simulink model "gm_stream_adaptation_model_fil"  (R2020b)
settings: Solver=FixedStepDiscrete  StartTime=0.0  StopTime=2  RelTol=1e-3
values from neighbouring files (symbols this model uses):
  frame = [frame zeros(num_of_pad_bits, 1)]    [pad_and_scramble.m]    (also in pad_and_scramble_test.m = randi([0 1], Kbch, 1); scrambler.m = in_frame)
libraries: simulink x3, hdlsllib x2, whdlio x1, fillib x1
settings Model: Creator=wardo  LastModifiedBy=EFlores
settings DataIOCC: LimitDataPoints=on  SaveOutput=off  SaveTime=off
settings OptimizationCC: BlockReduction=off  ConditionallyExecuteInputs=off  DefaultParameterBehavior=Inlined  LifeSpan=inf
settings DebuggingCC: AlgebraicLoopMsg=error  InheritedTsInSrcMsg=none  SingleTaskRateTransMsg=error  AllowSymbolicDim=off  StrictBusMsg=ErrorOnBusTreatedAsVector  SFUnexpectedBacktrackingDiag=warning  SFNoUnconditionalDefaultTransitionDiag=warning  SFExecutionAtInitializationDiag=none  ArithmeticOperatorsInVariantConditions=warning
settings HardwareCC: ProdBitPerPointer=32  ProdBitPerSizeT=32  ProdBitPerPtrDiffT=32  ProdLargestAtomicFloat=None  ProdIntDivRoundTo=Undefined  ProdEndianess=Unspecified  ProdWordSize=32  ProdHWDeviceType=ASIC/FPGA->ASIC/FPGA  ProdEqTarget=off
settings SFSimCC: SimUseLocalCustomCode=off  CustomCodeUndefinedFunction=UseInterfaceOnly
settings RTWCC: RTWUseLocalCustomCode=off
settings CodeAppCC: StateflowObjectComments=on
settings GRTTargetCC: TargetLangStandard=C89/C90 (ANSI)
settings ConfigComp: CovScope=ReferencedModels  CovMetricSettings=dw  CovSaveCumulativeToWorkspaceVar=on  CovSaveSingleToWorkspaceVar=on  CovExternalEMLEnable=off  CovSFcnEnable=off

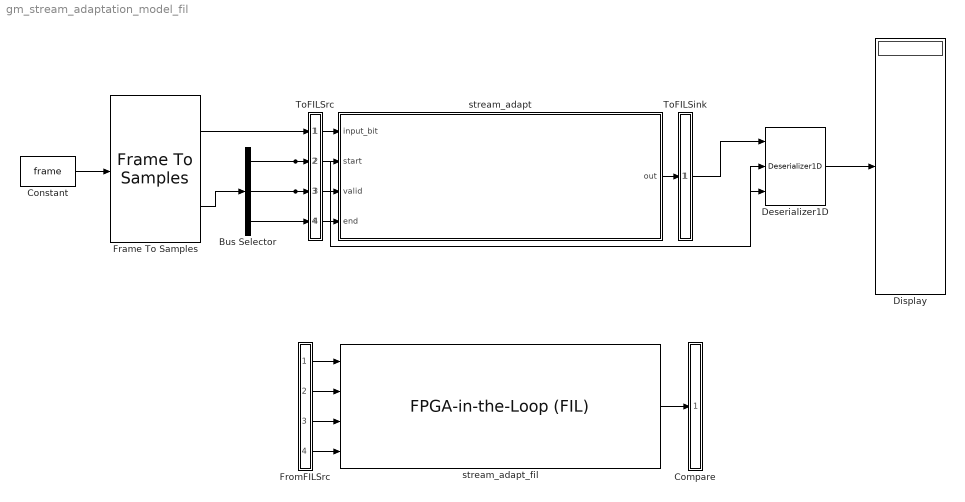
== system gm_stream_adaptation_model_fil ==
  Bus Selector : BusSelector  OutputSignals=start,valid,end
  Compare : Subsystem
      mask Display: disp('')
  Constant : Constant  Value=frame  OutDataTypeStr=fixdt(1,16)  SampleTime=1
  Deserializer1D : hdlsllib/HDL Operations/Deserializer1D  Ratio=48408  IdleCycles=0  InitialCondition=0  startIn=on  validIn=on  validOut=off  inputDataDimensions=-1  inputSampleTime=-1  inputSignalType=auto
      settings: SourceProductBaseCode=SL
  Display : Display
  Frame To Samples : whdlio/Frame To Samples  InterSampleIdleCycles=0  InterFrameIdleCycles=0  OutputSize=1  InterleaveSamples=off
      settings: SourceProductBaseCode=LH
  FromFILSrc : Subsystem
      mask Display: disp('')
  ToFILSink : Subsystem
      mask Display: disp('')
  ToFILSrc : Subsystem
      mask Display: disp('')
  stream_adapt : Subsystem
  stream_adapt_fil : fillib/FPGA-in-the-Loop (FIL)  ForceInterfaceUpdate=0.85357
      settings: SourceProductBaseCode=ES,HD
  wires:
  Constant/1 -> Frame To Samples/1
  Frame To Samples/2 -> Bus Selector/1
  Bus Selector/1 -> Deserializer1D/2, ToFILSrc/2(in2)
  Bus Selector/2 -> Deserializer1D/3, ToFILSrc/3(in3)
  Deserializer1D/1 -> Display/1
  ToFILSrc/1(out1) -> stream_adapt/1(input_bit)
  ToFILSrc/2(out2) -> stream_adapt/2(start)
  ToFILSrc/3(out3) -> stream_adapt/3(valid)
  ToFILSrc/4(out4) -> stream_adapt/4(end)
  stream_adapt/1(out) -> ToFILSink/1(in1)
  Frame To Samples/1 -> ToFILSrc/1(in1)
  Bus Selector/3 -> ToFILSrc/4(in4)
  ToFILSink/1(out1) -> Deserializer1D/1
  FromFILSrc/1(out1) -> stream_adapt_fil/1
  FromFILSrc/2(out2) -> stream_adapt_fil/2
  FromFILSrc/3(out3) -> stream_adapt_fil/3
  FromFILSrc/4(out4) -> stream_adapt_fil/4
  stream_adapt_fil/1 -> Compare/1(in1)

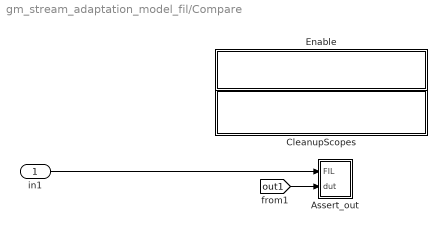
== system gm_stream_adaptation_model_fil/Compare ==
  in1 : Inport
  Assert_out : Subsystem
  CleanupScopes : Subsystem
      settings: OpenFcn=|
      | blkName = gcb; %self block
      | idx = regexp(blkName, '/CleanupScopes$', 'once');
      | blkParent = blkName(1:idx-1);
      | blks=find_system(blkParent, 'LookUnderMasks', 'all','blocktype', 'Scope');
      | for itr = 1:length(blks)
      | 	 hScopeCfg = get_param(blks{itr},'ScopeConfiguration');
      | 	 hScopeCfg.Visible = ~ hScopeCfg.Visible;
      | end
      | drawnow;
      mask Display: fprintf(message('hdlcoder:cosim:vnl_dblclick').getString());
  Enable : Subsystem
      settings: OpenFcn=|
      | blkName = gcb;
      | idx = regexp(blkName, '/Enable$', 'once');
      | blkParent = blkName(1:idx-1);
      | blks=find_system(blkParent, 'LookUnderMasks', 'all','blocktype', 'Assertion');
      | e = get_param(blks{1}, 'Enabled');
      | if strcmp(e, 'on'), f= 'off';, else, f = 'on';, end
      | for ii=1:length(blks), set_param(blks{ii}, 'Enabled', f);, end
      | set_param(gcb, 'MaskDisplay',['fprintf(message(''hdlcoder:cosim:vnl_dblclick_assertions'',','''',upper(e),'''',').getString())']);
      mask Display: fprintf(message('hdlcoder:cosim:vnl_dblclick_assertions','OFF').getString());
  wires:
  in1/1 -> Assert_out/1(FIL)
  [out1] -> Assert_out/2(dut)

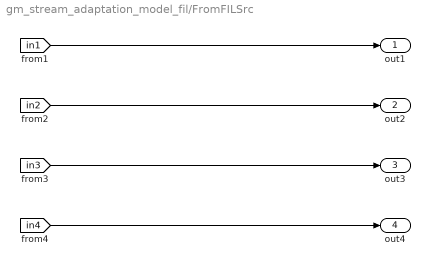
== system gm_stream_adaptation_model_fil/FromFILSrc ==
  out1 : Outport
  out2 : Outport  Port=2
  out3 : Outport  Port=3
  out4 : Outport  Port=4
  wires:
  [in1] -> out1/1
  [in2] -> out2/1
  [in3] -> out3/1
  [in4] -> out4/1

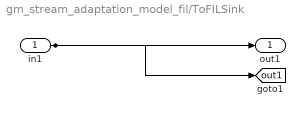
== system gm_stream_adaptation_model_fil/ToFILSink ==
  in1 : Inport
  out1 : Outport
  tag scope: out1=global
  wires:
  in1/1 -> out1/1, [out1]

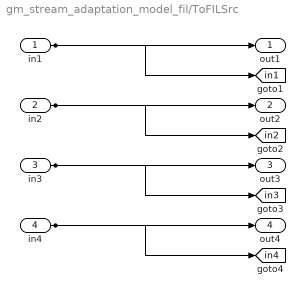
== system gm_stream_adaptation_model_fil/ToFILSrc ==
  in1 : Inport
  in2 : Inport  Port=2
  in3 : Inport  Port=3
  in4 : Inport  Port=4
  out1 : Outport
  out2 : Outport  Port=2
  out3 : Outport  Port=3
  out4 : Outport  Port=4
  tag scope: in1=global, in2=global, in3=global, in4=global
  wires:
  in1/1 -> out1/1, [in1]
  in2/1 -> out2/1, [in2]
  in3/1 -> out3/1, [in3]
  in4/1 -> out4/1, [in4]

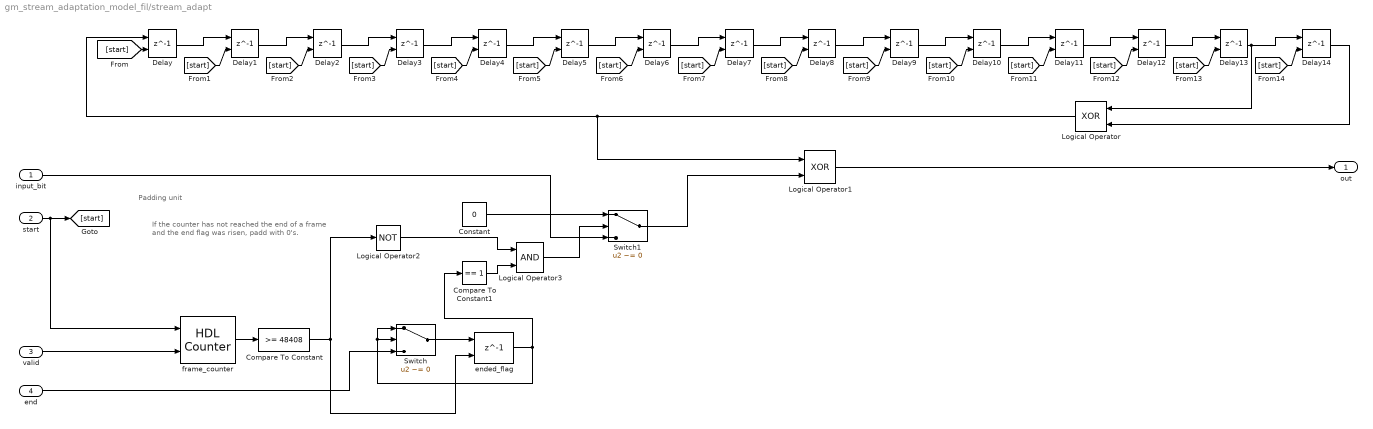
== system gm_stream_adaptation_model_fil/stream_adapt ==
  note: Padding unit
  note: If the counter has not reached the end of a frame and the end flag was risen,
      | padd with 0's.
  input_bit : Inport
  start : Inport  Port=2
  valid : Inport  Port=3
  end : Inport  Port=4
  Compare To Constant : simulink/Logic and Bit Operations/Compare To Constant  relop=>=  const=48408  OutDataTypeStr=boolean
  Compare To Constant1 : simulink/Logic and Bit Operations/Compare To Constant  relop===  const=1  OutDataTypeStr=boolean
  Constant : Constant  Value=0  OutDataTypeStr=fixdt(0,1)  SampleTime=-1
  Delay{,3,5,7} (4 alike) : Delay  DelayLength=1  InitialCondition=1  ExternalReset=Level
      settings: InputPortMap=u0,r5
  Delay{1..2,4,6,8..14} (11 alike) : Delay  DelayLength=1  ExternalReset=Level
      settings: InputPortMap=u0,r5
  Logical Operator : Logic  Operator=XOR  IconShape=distinctive  AllPortsSameDT=off  OutDataTypeStr=boolean
  Logical Operator1 : Logic  Operator=XOR  IconShape=distinctive  AllPortsSameDT=off  OutDataTypeStr=boolean
  Logical Operator2 : Logic  Operator=NOT  IconShape=distinctive  AllPortsSameDT=off  OutDataTypeStr=boolean
  Logical Operator3 : Logic  IconShape=distinctive  AllPortsSameDT=off  OutDataTypeStr=boolean
  Switch : Switch  Criteria=u2 ~= 0  OutDataTypeStr=boolean
  Switch1 : Switch  Criteria=u2 ~= 0
  ended_flag : Delay  DelayLength=1  ExternalReset=Level
      settings: InputPortMap=u0,r5
  frame_counter : hdlsllib/Sources/HDL Counter  CountType=Count limited  CountInit=0  CountStep=1  CountMax=48408  CountFromType=Initial value  CountFrom=0  CountResetPort=on  CountLoadPort=off  CountEnbPort=on  CountDirPort=off  CountDataType=Unsigned  CountWordLen=16  CountFracLen=0  CountSampTime=1
  out : Outport  VectorParamsAs1DForOutWhenUnconnected=off
  wires:
  Delay/1 -> Delay1/1
  Logical Operator/1 -> Delay/1, Logical Operator1/1
  Logical Operator1/1 -> out/1
  start/1 -> frame_counter/1, [start]
  [start] -> Delay/2
  [start] -> Delay1/2
  Delay1/1 -> Delay2/1
  [start] -> Delay2/2
  Delay2/1 -> Delay3/1
  [start] -> Delay3/2
  Delay3/1 -> Delay4/1
  [start] -> Delay4/2
  Delay4/1 -> Delay5/1
  [start] -> Delay5/2
  Delay5/1 -> Delay6/1
  [start] -> Delay6/2
  Delay6/1 -> Delay7/1
  [start] -> Delay7/2
  Delay7/1 -> Delay8/1
  [start] -> Delay8/2
  Delay8/1 -> Delay9/1
  [start] -> Delay9/2
  Delay9/1 -> Delay10/1
  [start] -> Delay10/2
  Delay10/1 -> Delay11/1
  [start] -> Delay11/2
  Delay11/1 -> Delay12/1
  [start] -> Delay12/2
  Delay12/1 -> Delay13/1
  [start] -> Delay13/2
  Delay13/1 -> Logical Operator/1, Delay14/1
  [start] -> Delay14/2
  Delay14/1 -> Logical Operator/2
  valid/1 -> frame_counter/2
  frame_counter/1 -> Compare To Constant/1
  Compare To Constant/1 -> ended_flag/2, Logical Operator2/1
  Switch/1 -> ended_flag/1
  end/1 -> Switch/3
  ended_flag/1 -> Switch/1, Switch/2, Compare To Constant1/1
  Compare To Constant1/1 -> Logical Operator3/2
  Logical Operator3/1 -> Switch1/2
  Logical Operator2/1 -> Logical Operator3/1
  Switch1/1 -> Logical Operator1/2
  input_bit/1 -> Switch1/3
  Constant/1 -> Switch1/1

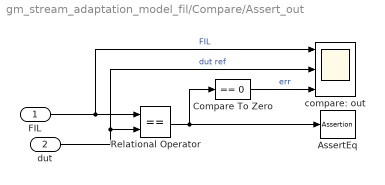
== system gm_stream_adaptation_model_fil/Compare/Assert_out ==
  FIL : Inport
  dut : Inport  Port=2
  AssertEq : Assertion  StopWhenAssertionFail=off
  Compare To Zero : simulink/Logic and Bit Operations/Compare To Zero  relop===  OutDataTypeStr=boolean
  Relational Operator : RelationalOperator  Operator===  OutDataTypeStr=boolean  RndMeth=Nearest
  compare: out : Scope  NumInputPorts=3
  wires:
  Compare To Zero/1 -> compare: out/3  "err"
  Relational Operator/1 -> Compare To Zero/1, AssertEq/1
  FIL/1 -> compare: out/1, Relational Operator/1  "FIL"
  dut/1 -> compare: out/2, Relational Operator/2  "dut ref"

== system gm_stream_adaptation_model_fil/Compare/CleanupScopes ==

== system gm_stream_adaptation_model_fil/Compare/Enable ==
